simulink model "sim_LQR_mul"  (R2015a)
settings: Solver=ode4  StartTime=0.  StopTime=10  FixedStep=Ts  MaxStep=0.005  RelTol=1e-3
values from neighbouring files (symbols this model uses):
  Alpha = pi/4    (= 0.785398163397)    [lqr_control_simple.m]
  Beta = 0    [lqr_control_simple.m]
  K_tot = dlqr(dsys.a, dsys.b, Q, R)    [lqr_control_simple.m]
undefined symbols (not defined in the file or in its folder): C11a, G21a, M11, M21a, M21b, M22, rk, rw, Ts
libraries: simulink x2
settings Model: CovSFcnEnable=off  Creator=THANH DANH  LastModifiedBy=desti
settings DebuggingCC: SolverPrmCheckMsg=warning

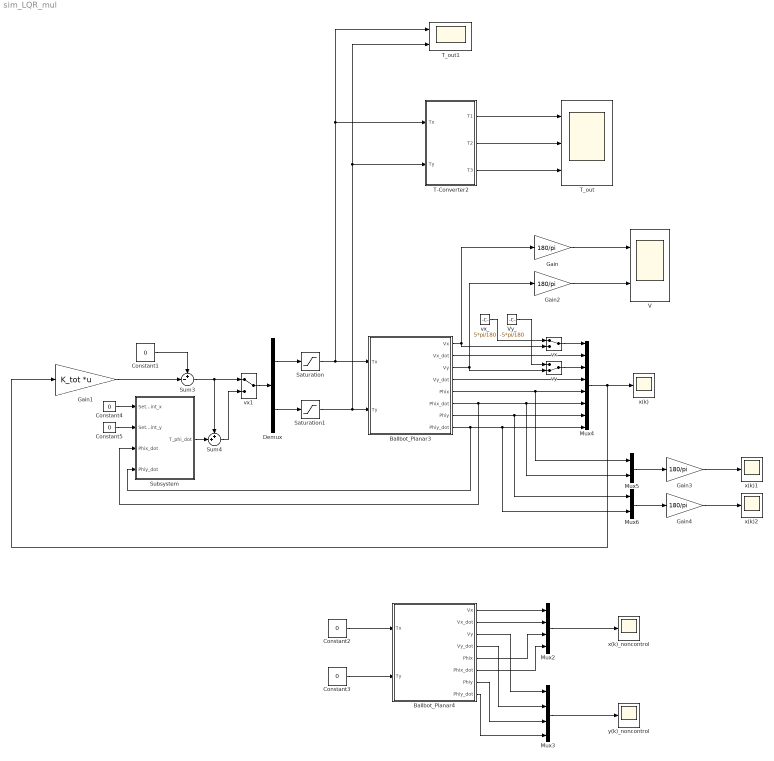
== system sim_LQR_mul ==
  Ballbot_Planar3 : Subsystem
  Ballbot_Planar4 : Subsystem
  Constant{1..5} (5 alike) : Constant  Value=0
  Demux : Demux  Outputs=2
  Gain{,2..4} (4 alike) : Gain  Gain=180/pi
  Gain1 : Gain  Gain=K_tot  Multiplication=Matrix(K*u)
  Mux2 : Mux
  Mux3 : Mux
  Mux4 : Mux  Inputs=8
  Mux5 : Mux  Inputs=2
  Mux6 : Mux  Inputs=2
  Saturation : Saturate  UpperLimit=5.5  LowerLimit=-5.5
  Saturation1 : Saturate  UpperLimit=5.5  LowerLimit=-5.5
  Subsystem : Subsystem
  Sum3 : Sum  Inputs=+-|
  Sum4 : Sum  Inputs=++|
  T-Converter2 : Subsystem
  T_out : Scope  NumInputPorts=3
      settings: TimeRange=1  YMin=0~-5~-5  YMax=0.09~5~5  SaveName=Vx4
  T_out1 : Scope  NumInputPorts=2
      settings: TimeRange=1  YMin=0~-5  YMax=0.09~5  SaveName=Txy
  V : Scope  NumInputPorts=2
      settings: TimeRange=1  YMin=0~-5  YMax=0.09~5  SaveName=V_mul
  Vy_ : Constant  Value=-5*pi/180
  vx : ManualSwitch
  vx1 : ManualSwitch
  vx_ : Constant  Value=5*pi/180
  vy : ManualSwitch  CurrentSetting=0
  x(k) : Scope
      settings: TimeRange=1  YMin=0  YMax=0.09  SaveName=Vx
  x(k)1 : Scope
      settings: TimeRange=1  YMin=0  YMax=0.09  SaveName=Vx3
  x(k)2 : Scope
      settings: TimeRange=1  YMin=0  YMax=0.09  SaveName=Vx5
  x(k)_noncontrol : Scope
      settings: TimeRange=1  YMin=0  YMax=0.09  SaveName=Vx1
  y(k)_noncontrol : Scope
      settings: TimeRange=1  YMin=0  YMax=0.09  SaveName=Vx2
  wires:
  Constant1/1 -> Sum3/1
  Mux4/1 -> x(k)/1, Gain1/1
  Gain1/1 -> Sum3/2
  Demux/1 -> Saturation/1
  Demux/2 -> Saturation1/1
  Ballbot_Planar4/5(Phix) -> Mux2/3
  Ballbot_Planar4/6(Phix_dot) -> Mux2/4
  Mux2/1 -> x(k)_noncontrol/1
  Constant2/1 -> Ballbot_Planar4/1(Tx)
  Ballbot_Planar4/1(Vx) -> Mux2/1
  Ballbot_Planar4/2(Vx_dot) -> Mux2/2
  Ballbot_Planar4/3(Vy) -> Mux3/1
  Ballbot_Planar4/4(Vy_dot) -> Mux3/2
  Ballbot_Planar4/7(Phiy) -> Mux3/3
  Ballbot_Planar4/8(Phiy_dot) -> Mux3/4
  Mux3/1 -> y(k)_noncontrol/1
  T-Converter2/1(T1) -> T_out/1
  T-Converter2/2(T2) -> T_out/2
  T-Converter2/3(T3) -> T_out/3
  Constant3/1 -> Ballbot_Planar4/2(Ty)
  Ballbot_Planar3/1(Vx) -> Gain/1, vx/2
  Ballbot_Planar3/2(Vx_dot) -> Mux4/2
  Ballbot_Planar3/3(Vy) -> Gain2/1, vy/2
  Ballbot_Planar3/4(Vy_dot) -> Mux4/4
  Ballbot_Planar3/5(Phix) -> Mux5/1, Mux4/5
  Ballbot_Planar3/6(Phix_dot) -> Subsystem/3(Phix_dot), Mux5/2, Mux4/6
  Ballbot_Planar3/7(Phiy) -> Mux6/1, Mux4/7
  Ballbot_Planar3/8(Phiy_dot) -> Subsystem/4(Phiy_dot), Mux6/2, Mux4/8
  vy/1 -> Mux4/3
  vx/1 -> Mux4/1
  vx_/1 -> vx/1
  Vy_/1 -> vy/1
  Sum3/1 -> Sum4/1, vx1/1
  Mux5/1 -> Gain3/1
  Mux6/1 -> Gain4/1
  vx1/1 -> Demux/1
  Gain/1 -> V/1
  Gain2/1 -> V/2
  Constant4/1 -> Subsystem/1(Set_point_x)
  Constant5/1 -> Subsystem/2(Set_point_y)
  Subsystem/1(T_phi_dot) -> Sum4/2
  Sum4/1 -> vx1/2
  Gain3/1 -> x(k)1/1
  Gain4/1 -> x(k)2/1
  Saturation/1 -> Ballbot_Planar3/1(Tx), T-Converter2/1(Tx), T_out1/1
  Saturation1/1 -> Ballbot_Planar3/2(Ty), T-Converter2/2(Ty), T_out1/2

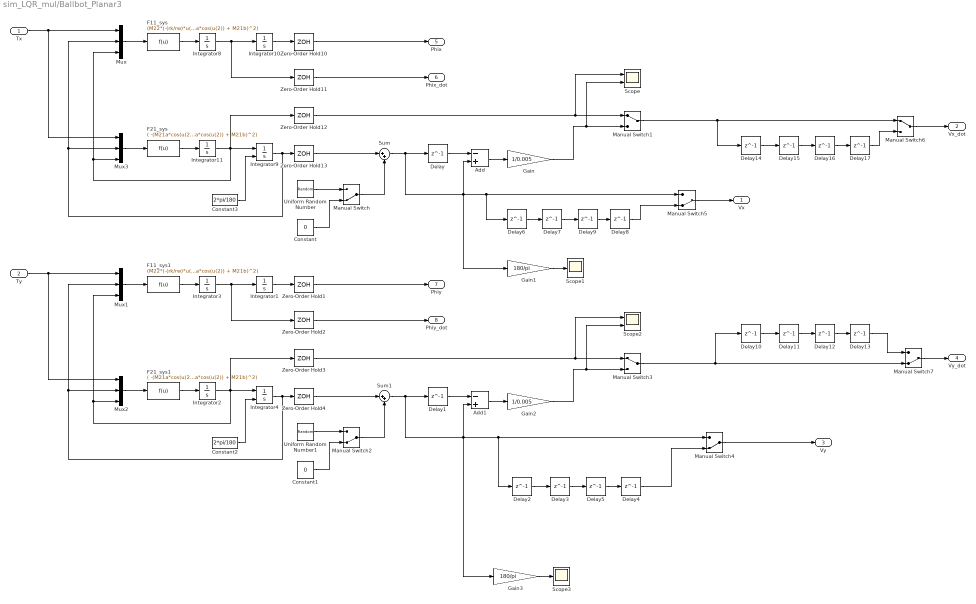
== system sim_LQR_mul/Ballbot_Planar3 ==
  Tx : Inport
  Ty : Inport  Port=2
  Add : Sum  Inputs=-+
  Add1 : Sum  Inputs=-+
  Constant : Constant  Value=0
  Constant1 : Constant  Value=0
  Constant2 : Constant  Value=2*pi/180
  Constant3 : Constant  Value=2*pi/180
  Delay{,1..17} (18 alike) : Delay  DelayLength=1
  F11_sys : Fcn  Expr=(M22*(-(rk/rw)*u(1) - C11a*sin(u(2))*(u(3))^2) - (M21a*cos(u(2)) + M21b)*(-(rk/rw)*u(1) - G21a*sin(u(2)))) / (M11*M22 - (M21a*cos(u(2)) + M21b)^2)
  F11_sys1 : Fcn  Expr=(M22*(-(rk/rw)*u(1) - C11a*sin(u(2))*(u(3))^2) - (M21a*cos(u(2)) + M21b)*(-(rk/rw)*u(1) - G21a*sin(u(2)))) / (M11*M22 - (M21a*cos(u(2)) + M21b)^2)
  F21_sys : Fcn  Expr=( -(M21a*cos(u(2)) + M21b)*(-(rk/rw)*u(1) - C11a*sin(u(2))*(u(3))^2) + M11*(-(rk/rw)*u(1) - G21a*sin(u(2))) ) / (M11*M22 - (M21a*cos(u(2)) + M21b)^2)
  F21_sys1 : Fcn  Expr=( -(M21a*cos(u(2)) + M21b)*(-(rk/rw)*u(1) - C11a*sin(u(2))*(u(3))^2) + M11*(-(rk/rw)*u(1) - G21a*sin(u(2))) ) / (M11*M22 - (M21a*cos(u(2)) + M21b)^2)
  Gain : Gain  Gain=1/0.005
  Gain1 : Gain  Gain=180/pi
  Gain2 : Gain  Gain=1/0.005
  Gain3 : Gain  Gain=180/pi
  Integrator{1..3,8,10..11} (6 alike) : Integrator
  Integrator4 : Integrator  InitialConditionSource=external
  Integrator9 : Integrator  InitialConditionSource=external
  Manual Switch{,2,4..5,7} (5 alike) : ManualSwitch  CurrentSetting=0
  Manual Switch1 : ManualSwitch
  Manual Switch3 : ManualSwitch
  Manual Switch6 : ManualSwitch
  Mux{,1..3} (4 alike) : Mux  Inputs=3
  Scope : Scope  NumInputPorts=2
      settings: YMin=-5~-5  YMax=5~5  SaveName=ScopeData6
  Scope1 : Scope
      settings: SaveName=ScopeData7
  Scope2 : Scope  NumInputPorts=2
      settings: YMin=-5~-5  YMax=5~5
  Scope3 : Scope
  Sum : Sum  Inputs=|++
  Sum1 : Sum  Inputs=|++
  Uniform Random Number : UniformRandomNumber  Minimum=-0.2*pi/180  Maximum=0.2*pi/180  SampleTime=Ts
  Uniform Random Number1 : UniformRandomNumber  Minimum=-0.2*pi/180  Maximum=0.2*pi/180  SampleTime=Ts
  Zero-Order Hold{1..4,10..13} (8 alike) : ZeroOrderHold  SampleTime=Ts
  Vx : Outport
  Vx_dot : Outport  Port=2
  Vy : Outport  Port=3
  Vy_dot : Outport  Port=4
  Phix : Outport  Port=5
  Phix_dot : Outport  Port=6
  Phiy : Outport  Port=7
  Phiy_dot : Outport  Port=8
  wires:
  Integrator11/1 -> Integrator9/1, Zero-Order Hold12/1, Mux/3, Mux3/3
  Integrator8/1 -> Integrator10/1, Zero-Order Hold11/1
  Integrator10/1 -> Zero-Order Hold10/1
  Integrator9/1 -> Zero-Order Hold13/1, Mux/2, Mux3/2
  F21_sys/1 -> Integrator11/1
  Mux3/1 -> F21_sys/1
  Mux/1 -> F11_sys/1
  F11_sys/1 -> Integrator8/1
  Tx/1 -> Mux3/1, Mux/1
  Constant3/1 -> Integrator9/2
  Zero-Order Hold10/1 -> Phix/1
  Zero-Order Hold11/1 -> Phix_dot/1
  Zero-Order Hold12/1 -> Scope/1, Manual Switch1/1
  Zero-Order Hold13/1 -> Sum/1
  Sum/1 -> Delay/1, Add/2, Delay6/1, Manual Switch5/1, Gain1/1
  Delay/1 -> Add/1
  Add/1 -> Gain/1
  Gain/1 -> Scope/2, Manual Switch1/2
  Uniform Random Number/1 -> Manual Switch/1
  Constant/1 -> Manual Switch/2
  Manual Switch/1 -> Sum/2
  Gain1/1 -> Scope1/1
  Integrator2/1 -> Integrator4/1, Zero-Order Hold3/1, Mux1/3, Mux2/3
  Integrator3/1 -> Integrator1/1, Zero-Order Hold2/1
  Integrator1/1 -> Zero-Order Hold1/1
  Integrator4/1 -> Zero-Order Hold4/1, Mux1/2, Mux2/2
  F21_sys1/1 -> Integrator2/1
  Mux2/1 -> F21_sys1/1
  Mux1/1 -> F11_sys1/1
  F11_sys1/1 -> Integrator3/1
  Ty/1 -> Mux2/1, Mux1/1
  Constant2/1 -> Integrator4/2
  Zero-Order Hold1/1 -> Phiy/1
  Zero-Order Hold2/1 -> Phiy_dot/1
  Zero-Order Hold3/1 -> Scope2/1, Manual Switch3/1
  Zero-Order Hold4/1 -> Sum1/1
  Sum1/1 -> Delay1/1, Manual Switch4/1, Delay2/1, Gain3/1, Add1/2
  Delay1/1 -> Add1/1
  Add1/1 -> Gain2/1
  Gain2/1 -> Scope2/2, Manual Switch3/2
  Uniform Random Number1/1 -> Manual Switch2/1
  Constant1/1 -> Manual Switch2/2
  Manual Switch2/1 -> Sum1/2
  Gain3/1 -> Scope3/1
  Manual Switch4/1 -> Vy/1
  Delay2/1 -> Delay3/1
  Delay3/1 -> Delay5/1
  Delay6/1 -> Delay7/1
  Delay7/1 -> Delay9/1
  Manual Switch5/1 -> Vx/1
  Delay10/1 -> Delay11/1
  Delay11/1 -> Delay12/1
  Delay12/1 -> Delay13/1
  Delay14/1 -> Delay15/1
  Delay15/1 -> Delay16/1
  Delay16/1 -> Delay17/1
  Manual Switch6/1 -> Vx_dot/1
  Manual Switch1/1 -> Delay14/1, Manual Switch6/1
  Delay17/1 -> Manual Switch6/2
  Manual Switch7/1 -> Vy_dot/1
  Manual Switch3/1 -> Delay10/1, Manual Switch7/2
  Delay13/1 -> Manual Switch7/1
  Delay4/1 -> Manual Switch4/2
  Delay5/1 -> Delay4/1
  Delay8/1 -> Manual Switch5/2
  Delay9/1 -> Delay8/1

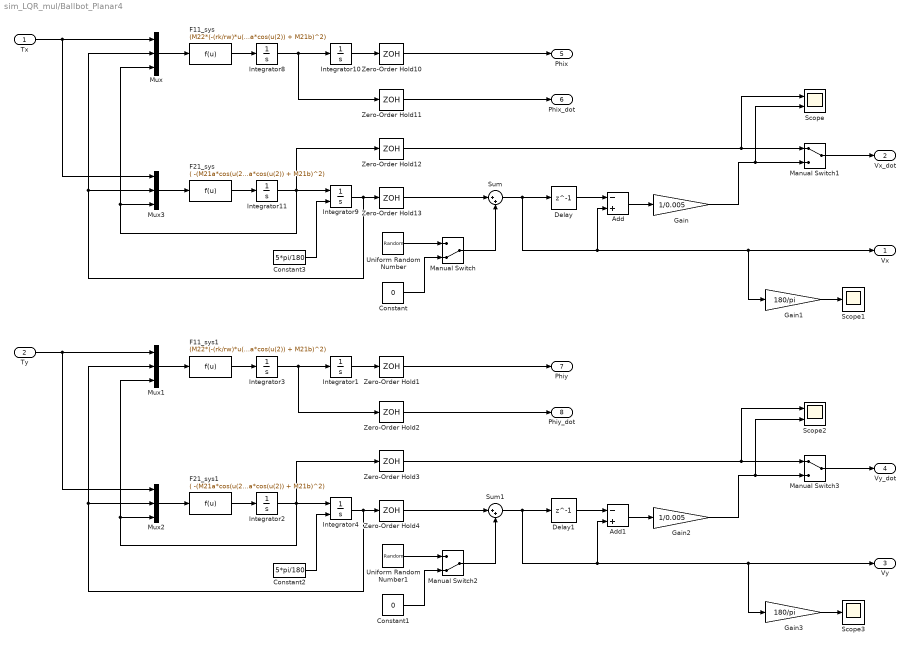
== system sim_LQR_mul/Ballbot_Planar4 ==
  Tx : Inport
  Ty : Inport  Port=2
  Add : Sum  Inputs=-+
  Add1 : Sum  Inputs=-+
  Constant : Constant  Value=0
  Constant1 : Constant  Value=0
  Constant2 : Constant  Value=5*pi/180
  Constant3 : Constant  Value=5*pi/180
  Delay : Delay  DelayLength=1
  Delay1 : Delay  DelayLength=1
  F11_sys : Fcn  Expr=(M22*(-(rk/rw)*u(1) - C11a*sin(u(2))*(u(3))^2) - (M21a*cos(u(2)) + M21b)*(-(rk/rw)*u(1) - G21a*sin(u(2)))) / (M11*M22 - (M21a*cos(u(2)) + M21b)^2)
  F11_sys1 : Fcn  Expr=(M22*(-(rk/rw)*u(1) - C11a*sin(u(2))*(u(3))^2) - (M21a*cos(u(2)) + M21b)*(-(rk/rw)*u(1) - G21a*sin(u(2)))) / (M11*M22 - (M21a*cos(u(2)) + M21b)^2)
  F21_sys : Fcn  Expr=( -(M21a*cos(u(2)) + M21b)*(-(rk/rw)*u(1) - C11a*sin(u(2))*(u(3))^2) + M11*(-(rk/rw)*u(1) - G21a*sin(u(2))) ) / (M11*M22 - (M21a*cos(u(2)) + M21b)^2)
  F21_sys1 : Fcn  Expr=( -(M21a*cos(u(2)) + M21b)*(-(rk/rw)*u(1) - C11a*sin(u(2))*(u(3))^2) + M11*(-(rk/rw)*u(1) - G21a*sin(u(2))) ) / (M11*M22 - (M21a*cos(u(2)) + M21b)^2)
  Gain : Gain  Gain=1/0.005
  Gain1 : Gain  Gain=180/pi
  Gain2 : Gain  Gain=1/0.005
  Gain3 : Gain  Gain=180/pi
  Integrator{1..3,8,10..11} (6 alike) : Integrator
  Integrator4 : Integrator  InitialConditionSource=external
  Integrator9 : Integrator  InitialConditionSource=external
  Manual Switch : ManualSwitch  CurrentSetting=0
  Manual Switch1 : ManualSwitch
  Manual Switch2 : ManualSwitch  CurrentSetting=0
  Manual Switch3 : ManualSwitch
  Mux{,1..3} (4 alike) : Mux  Inputs=3
  Scope : Scope  NumInputPorts=2
      settings: YMin=-5~-5  YMax=5~5  SaveName=ScopeData6
  Scope1 : Scope
      settings: SaveName=ScopeData7
  Scope2 : Scope  NumInputPorts=2
      settings: YMin=-5~-5  YMax=5~5
  Scope3 : Scope
  Sum : Sum  Inputs=|++
  Sum1 : Sum  Inputs=|++
  Uniform Random Number : UniformRandomNumber  Minimum=-0.2*pi/180  Maximum=0.2*pi/180  SampleTime=Ts
  Uniform Random Number1 : UniformRandomNumber  Minimum=-0.2*pi/180  Maximum=0.2*pi/180  SampleTime=Ts
  Zero-Order Hold{1..4,10..13} (8 alike) : ZeroOrderHold  SampleTime=Ts
  Vx : Outport
  Vx_dot : Outport  Port=2
  Vy : Outport  Port=3
  Vy_dot : Outport  Port=4
  Phix : Outport  Port=5
  Phix_dot : Outport  Port=6
  Phiy : Outport  Port=7
  Phiy_dot : Outport  Port=8
  wires:
  Gain3/1 -> Scope3/1
  Manual Switch3/1 -> Vy_dot/1
  Manual Switch2/1 -> Sum1/2
  Constant1/1 -> Manual Switch2/2
  Uniform Random Number1/1 -> Manual Switch2/1
  Gain2/1 -> Manual Switch3/2, Scope2/2
  Add1/1 -> Gain2/1
  Delay1/1 -> Add1/1
  Sum1/1 -> Add1/2, Vy/1, Gain3/1, Delay1/1
  Zero-Order Hold4/1 -> Sum1/1
  Zero-Order Hold3/1 -> Manual Switch3/1, Scope2/1
  Zero-Order Hold2/1 -> Phiy_dot/1
  Zero-Order Hold1/1 -> Phiy/1
  Constant2/1 -> Integrator4/2
  Ty/1 -> Mux1/1, Mux2/1
  F11_sys1/1 -> Integrator3/1
  Mux1/1 -> F11_sys1/1
  Mux2/1 -> F21_sys1/1
  F21_sys1/1 -> Integrator2/1
  Integrator4/1 -> Mux2/2, Mux1/2, Zero-Order Hold4/1
  Integrator1/1 -> Zero-Order Hold1/1
  Integrator3/1 -> Zero-Order Hold2/1, Integrator1/1
  Integrator2/1 -> Mux2/3, Mux1/3, Zero-Order Hold3/1, Integrator4/1
  Gain1/1 -> Scope1/1
  Manual Switch1/1 -> Vx_dot/1
  Manual Switch/1 -> Sum/2
  Constant/1 -> Manual Switch/2
  Uniform Random Number/1 -> Manual Switch/1
  Gain/1 -> Manual Switch1/2, Scope/2
  Add/1 -> Gain/1
  Delay/1 -> Add/1
  Sum/1 -> Add/2, Vx/1, Gain1/1, Delay/1
  Zero-Order Hold13/1 -> Sum/1
  Zero-Order Hold12/1 -> Manual Switch1/1, Scope/1
  Zero-Order Hold11/1 -> Phix_dot/1
  Zero-Order Hold10/1 -> Phix/1
  Constant3/1 -> Integrator9/2
  Tx/1 -> Mux/1, Mux3/1
  F11_sys/1 -> Integrator8/1
  Mux/1 -> F11_sys/1
  Mux3/1 -> F21_sys/1
  F21_sys/1 -> Integrator11/1
  Integrator9/1 -> Mux3/2, Mux/2, Zero-Order Hold13/1
  Integrator10/1 -> Zero-Order Hold10/1
  Integrator8/1 -> Zero-Order Hold11/1, Integrator10/1
  Integrator11/1 -> Mux3/3, Mux/3, Zero-Order Hold12/1, Integrator9/1

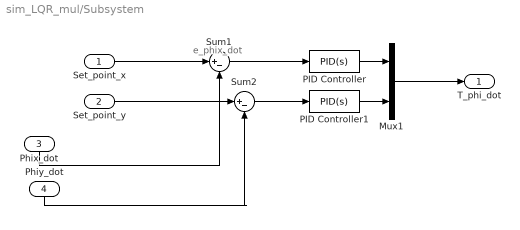
== system sim_LQR_mul/Subsystem ==
  note: e_phix_dot
  Set_point_x : Inport
  Set_point_y : Inport  Port=2
  Phix_dot : Inport  Port=3
  Phiy_dot : Inport  Port=4
  Mux1 : Mux  Inputs=2
  PID Controller : simulink/Continuous/PID Controller  Controller=PID  TimeDomain=Continuous-time  SampleTime=-1  IntegratorMethod=Forward Euler  FilterMethod=Forward Euler  Form=Parallel  UseFilter=on  ControllerParametersSource=internal  P=0.5  I=0.3  D=0  N=100  InitialConditionSource=internal  InitialConditionForIntegrator=0  InitialConditionForFilter=0  ExternalReset=none  LimitOutput=off  UpperSaturationLimit=inf  LowerSaturationLimit=-inf  LinearizeAsGain=on  AntiWindupMode=none  Kb=1  TrackingMode=off  Kt=1  PParamMin=[]  PParamMax=[]  IParamMin=[]  IParamMax=[]  DParamMin=[]  DParamMax=[]  NParamMin=[]  NParamMax=[]  KbParamMin=[]  KbParamMax=[]  KtParamMin=[]  KtParamMax=[]  POutMin=[]  POutMax=[]  IOutMin=[]  IOutMax=[]  DOutMin=[]  DOutMax=[]  NOutMin=[]  NOutMax=[]  KbOutMin=[]  KbOutMax=[]  KtOutMin=[]  KtOutMax=[]  IntegratorOutMin=[]  IntegratorOutMax=[]  FilterOutMin=[]  FilterOutMax=[]  SumOutMin=[]  SumOutMax=[]  SumI1OutMin=[]  SumI1OutMax=[]  SumI2OutMin=[]  SumI2OutMax=[]  SumI3OutMin=[]  SumI3OutMax=[]  SumDOutMin=[]  SumDOutMax=[]  SaturationOutMin=[]  SaturationOutMax=[]  IntegratorContinuousStateAttributes=''  IntegratorStateMustResolveToSignalObject=off  IntegratorRTWStateStorageClass=Auto  FilterContinuousStateAttributes=''  FilterStateMustResolveToSignalObject=off  FilterRTWStateStorageClass=Auto  DifferentiatorICPrevScaledInput=0  DifferentiatorOutMin=[]  DifferentiatorOutMax=[]
  PID Controller1 : simulink/Continuous/PID Controller  Controller=PID  TimeDomain=Continuous-time  SampleTime=-1  IntegratorMethod=Forward Euler  FilterMethod=Forward Euler  Form=Parallel  UseFilter=on  ControllerParametersSource=internal  P=0.5  I=0.3  D=0  N=100  InitialConditionSource=internal  InitialConditionForIntegrator=0  InitialConditionForFilter=0  ExternalReset=none  LimitOutput=off  UpperSaturationLimit=inf  LowerSaturationLimit=-inf  LinearizeAsGain=on  AntiWindupMode=none  Kb=1  TrackingMode=off  Kt=1  PParamMin=[]  PParamMax=[]  IParamMin=[]  IParamMax=[]  DParamMin=[]  DParamMax=[]  NParamMin=[]  NParamMax=[]  KbParamMin=[]  KbParamMax=[]  KtParamMin=[]  KtParamMax=[]  POutMin=[]  POutMax=[]  IOutMin=[]  IOutMax=[]  DOutMin=[]  DOutMax=[]  NOutMin=[]  NOutMax=[]  KbOutMin=[]  KbOutMax=[]  KtOutMin=[]  KtOutMax=[]  IntegratorOutMin=[]  IntegratorOutMax=[]  FilterOutMin=[]  FilterOutMax=[]  SumOutMin=[]  SumOutMax=[]  SumI1OutMin=[]  SumI1OutMax=[]  SumI2OutMin=[]  SumI2OutMax=[]  SumI3OutMin=[]  SumI3OutMax=[]  SumDOutMin=[]  SumDOutMax=[]  SaturationOutMin=[]  SaturationOutMax=[]  IntegratorContinuousStateAttributes=''  IntegratorStateMustResolveToSignalObject=off  IntegratorRTWStateStorageClass=Auto  FilterContinuousStateAttributes=''  FilterStateMustResolveToSignalObject=off  FilterRTWStateStorageClass=Auto  DifferentiatorICPrevScaledInput=0  DifferentiatorOutMin=[]  DifferentiatorOutMax=[]
  Sum1 : Sum  Inputs=|+-
  Sum2 : Sum  Inputs=|+-
  T_phi_dot : Outport
  wires:
  Sum1/1 -> PID Controller/1
  PID Controller1/1 -> Mux1/2
  Set_point_x/1 -> Sum1/1
  Set_point_y/1 -> Sum2/1
  Mux1/1 -> T_phi_dot/1
  PID Controller/1 -> Mux1/1
  Sum2/1 -> PID Controller1/1
  Phix_dot/1 -> Sum1/2
  Phiy_dot/1 -> Sum2/2

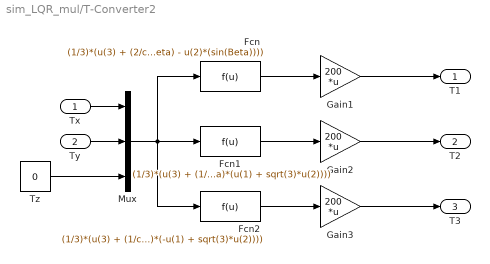
== system sim_LQR_mul/T-Converter2 ==
  Tx : Inport
  Ty : Inport  Port=2
  Fcn : Fcn  Expr=(1/3)*(u(3) + (2/cos(Alpha))*(u(1)*cos(Beta) - u(2)*(sin(Beta))))
  Fcn1 : Fcn  Expr=(1/3)*(u(3) + (1/cos(Alpha))*( sin(Beta)*((-sqrt(3))*u(1) + u(2)) - cos(Beta)*(u(1) + sqrt(3)*u(2))))
  Fcn2 : Fcn  Expr=(1/3)*(u(3) + (1/cos(Alpha))*( sin(Beta)*(sqrt(3)*u(1) + u(2)) + cos(Beta)*(-u(1) + sqrt(3)*u(2))))
  Gain1 : Gain  Gain=200  Multiplication=Matrix(K*u)
  Gain2 : Gain  Gain=200  Multiplication=Matrix(K*u)
  Gain3 : Gain  Gain=200  Multiplication=Matrix(K*u)
  Mux : Mux  Inputs=3
  Tz : Constant  Value=0
  T1 : Outport
  T2 : Outport  Port=2
  T3 : Outport  Port=3
  wires:
  Fcn/1 -> Gain1/1
  Fcn1/1 -> Gain2/1
  Fcn2/1 -> Gain3/1
  Tx/1 -> Mux/1
  Ty/1 -> Mux/2
  Mux/1 -> Fcn2/1, Fcn/1, Fcn1/1
  Tz/1 -> Mux/3
  Gain1/1 -> T1/1
  Gain2/1 -> T2/1
  Gain3/1 -> T3/1
